simulink library "ccb"  (Simulink 8.1)
settings: Solver=ode1  StartTime=0.0  StopTime=Inf  FixedStep=0.001  RelTol=1e-3
PostLoadFcn:
  | , if any(exist('dsrtsu_mdlpostloadfcn', 'file') == [2, 3, 6]), try dsrtsu_mdlpostloadfcn('Execute', bdroot); catch fprintf('Error in PostLoadFcn (dsrtsu_mdlpostloadfcn) for model "%s":\n %s\n', bdroot, lasterr); end, end,
settings Model: DSRTSU_INTERNAL_RTI_VER=450  DSRTSU_INTERNAL_RTI_TYPE=rti1401  RTICANMMDATA=struct('GeneralSetupData',struct('modelroot','D:\ELN150201_TAIWAN\trunk\AdasDragon\software\sw_development\arch\app\acc','generalsettings',struct('filesettings',struct('destfolder',struct('Name','RTICANMM_FILES','Check',1),'buildfolder',struct('Name','.','Check',1),'AbsDestfolder',struct('Name','D:\ELN150201_TAIWAN\trunk\AdasDragon\software\sw_development\arch\app\acc\RTICANMM_FILES'),'AbsBuildfolder',struct('Name','D:\ELN150201_TAIWAN\trunk\AdasDragon\software\sw_development\arch\app\acc'))),'options',struct('addpaths',1,'rmpaths',1,'addtrcexclusion',logical(1),'cannavigator',struct('checkmonitoring',0),'show_usrtrc',0,'use_usrtrc',0),'advanced',struct('options',[1 1 1 1 1 1 1 1 1 1 1 1 1 1 1 1 1 1 1 1 1 1 1 1 1 1 1 1 1 1 1 1 1 1 1 1 1 1 1 1 1 1 1 1 1 1 1 1 1 1 1 1 1 1 1 1 1 1 1 1 1 1 1 1 1 1 1 1 1 1 1 1 1 1 1 1 1 1 1 1 1 1 1 1 1 1 1 1 1 1 1 1 1 1 1 1 1 1 1 1]),'MPSetup',{{}},'modelname','ccb','block','ccb'))  DSRTSU_INTERNAL_RTIFPGA=40  Creator=AT015555  LastModifiedBy=AT015555

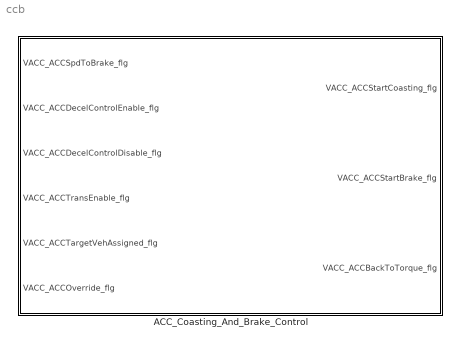
== system ccb ==
  ACC_Coasting_And_Brake_Control : Subsystem

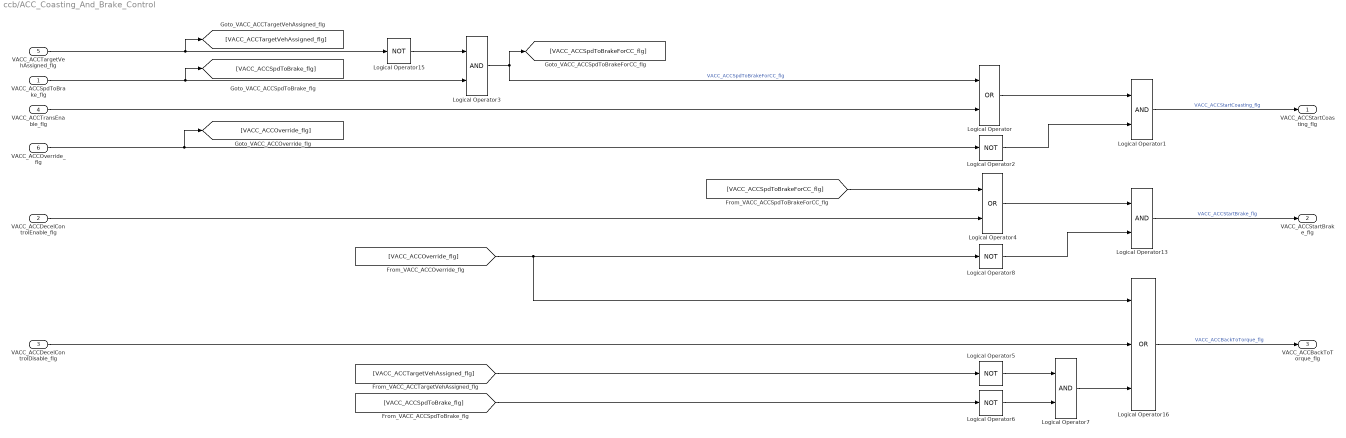
== system ccb/ACC_Coasting_And_Brake_Control ==
  VACC_ACCSpdToBrake_flg : Inport
  VACC_ACCDecelControlEnable_flg : Inport  Port=2
  VACC_ACCDecelControlDisable_flg : Inport  Port=3
  VACC_ACCTransEnable_flg : Inport  Port=4
  VACC_ACCTargetVehAssigned_flg : Inport  Port=5
  VACC_ACCOverride_flg : Inport  Port=6
  Logical Operator : Logic  Operator=OR  AllPortsSameDT=off  OutDataTypeStr=boolean
  Logical Operator{1,3,7,13} (4 alike) : Logic  AllPortsSameDT=off  OutDataTypeStr=boolean
  Logical Operator{2,5..6,8,15} (5 alike) : Logic  Operator=NOT  AllPortsSameDT=off  OutDataTypeStr=boolean
  Logical Operator16 : Logic  Operator=OR  Inputs=3  AllPortsSameDT=off  OutDataTypeStr=boolean
  Logical Operator4 : Logic  Operator=OR  AllPortsSameDT=off  OutDataTypeStr=boolean
  VACC_ACCStartCoasting_flg : Outport
  VACC_ACCStartBrake_flg : Outport  Port=2
  VACC_ACCBackToTorque_flg : Outport  Port=3
  wires:
  Logical Operator13/1 -> VACC_ACCStartBrake_flg/1  "VACC_ACCStartBrake_flg"
  Logical Operator16/1 -> VACC_ACCBackToTorque_flg/1  "VACC_ACCBackToTorque_flg"
  VACC_ACCOverride_flg/1 -> Logical Operator2/1, [VACC_ACCOverride_flg]
  Logical Operator1/1 -> VACC_ACCStartCoasting_flg/1  "VACC_ACCStartCoasting_flg"
  VACC_ACCTransEnable_flg/1 -> Logical Operator/2
  VACC_ACCSpdToBrake_flg/1 -> [VACC_ACCSpdToBrake_flg], Logical Operator3/2
  Logical Operator/1 -> Logical Operator1/1
  [VACC_ACCSpdToBrakeForCC_flg] -> Logical Operator4/1
  VACC_ACCDecelControlEnable_flg/1 -> Logical Operator4/2
  Logical Operator2/1 -> Logical Operator1/2
  [VACC_ACCOverride_flg] -> Logical Operator16/1, Logical Operator8/1
  Logical Operator4/1 -> Logical Operator13/1
  Logical Operator8/1 -> Logical Operator13/2
  VACC_ACCTargetVehAssigned_flg/1 -> [VACC_ACCTargetVehAssigned_flg], Logical Operator15/1
  Logical Operator15/1 -> Logical Operator3/1
  VACC_ACCDecelControlDisable_flg/1 -> Logical Operator16/2
  Logical Operator3/1 -> Logical Operator/1, [VACC_ACCSpdToBrakeForCC_flg]  "VACC_ACCSpdToBrakeForCC_flg"
  [VACC_ACCTargetVehAssigned_flg] -> Logical Operator5/1
  [VACC_ACCSpdToBrake_flg] -> Logical Operator6/1
  Logical Operator5/1 -> Logical Operator7/1
  Logical Operator6/1 -> Logical Operator7/2
  Logical Operator7/1 -> Logical Operator16/3
